simulink model "scc_ut"  (Simulink 8.1)
settings: Solver=FixedStepDiscrete  StartTime=0.0  StopTime=10  FixedStep=5E-3  RelTol=1e-3
PostLoadFcn:
  | , if any(exist('dsrtsu_mdlpostloadfcn', 'file') == [2, 3, 6]), try dsrtsu_mdlpostloadfcn('Execute', bdroot); catch fprintf('Error in PostLoadFcn (dsrtsu_mdlpostloadfcn) for model "%s":\n %s\n', bdroot, lasterr); end, end,
libraries: siltestlib x20, scc x1
settings Model: DSRTSU_INTERNAL_RTI_VER=450  DSRTSU_INTERNAL_RTI_TYPE=rti1401  RTICANMMDATA=struct('GeneralSetupData',struct('modelroot','D:\ELN150201_TAIWAN\trunk\AdasDragon\software\sw_development\arch\app\acc','generalsettings',struct('filesettings',struct('destfolder',struct('Name','RTICANMM_FILES','Check',1),'buildfolder',struct('Name','.','Check',1),'AbsDestfolder',struct('Name','D:\ELN150201_TAIWAN\trunk\AdasDragon\software\sw_development\arch\app\acc\RTICANMM_FILES'),'AbsBuildfolder',struct('Name','D:\ELN150201_TAIWAN\trunk\AdasDragon\software\sw_development\arch\app\acc'))),'options',struct('addpaths',1,'rmpaths',1,'addtrcexclusion',logical(1),'cannavigator',struct('checkmonitoring',0),'show_usrtrc',0,'use_usrtrc',0),'advanced',struct('options',[1 1 1 1 1 1 1 1 1 1 1 1 1 1 1 1 1 1 1 1 1 1 1 1 1 1 1 1 1 1 1 1 1 1 1 1 1 1 1 1 1 1 1 1 1 1 1 1 1 1 1 1 1 1 1 1 1 1 1 1 1 1 1 1 1 1 1 1 1 1 1 1 1 1 1 1 1 1 1 1 1 1 1 1 1 1 1 1 1 1 1 1 1 1 1 1 1 1 1 1]),'MPSetup',{{}},'modelname','scc_ut','block','scc_ut'))  DSRTSU_INTERNAL_RTIFPGA=40  Creator=AT015411  LastModifiedBy=AT015555  BufferReuse=off
settings DataIOCC: SignalLoggingSaveFormat=Dataset
settings OptimizationCC: BlockReduction=off  OptimizeBlockIOStorage=off  BufferReuse=off  ExpressionFolding=off  ExpressionDepthLimit=128  LocalBlockOutputs=off
settings DebuggingCC: FcnCallInpInsideContextMsg=EnableAllAsError
settings HardwareCC: ProdIntDivRoundTo=Zero  ProdEndianess=BigEndian  ProdHWDeviceType=Generic->Custom  TargetIntDivRoundTo=Zero  TargetEndianess=BigEndian  TargetHWDeviceType=Generic->Custom
settings RTWCC: SystemTargetFile=rti1005.tlc  MakeCommand=make_rti  TemplateMakefile=rti1005.tmf  Description=dSPACE DS1005 Hardware Platform  ProcessScript=rti1005_make_rtw_hook
settings STFCustomTargetCC: CodeReplacementLibrary=ANSI_C  ParMdlRefBuildCompliant=on  GeneratePreprocessorConditionals=Disable all  MatFileLogging=on  SystemTargetFile=rti1005.tlc
settings GRTTargetCC: CompOptLevelCompliant=off  ConcurrentExecutionCompliant=off  ExtModeMexFile=noextcomm
settings CustomProperty: DataType=RTWOptions_EnumType_C__Program Files (x86)_dSPACE RCPHIL 2014-B_MATLAB_RTI_RTI1401_TLC_rti1005_1InitialSimState  Value=RUN
settings EnumStrPairs: String=RUN

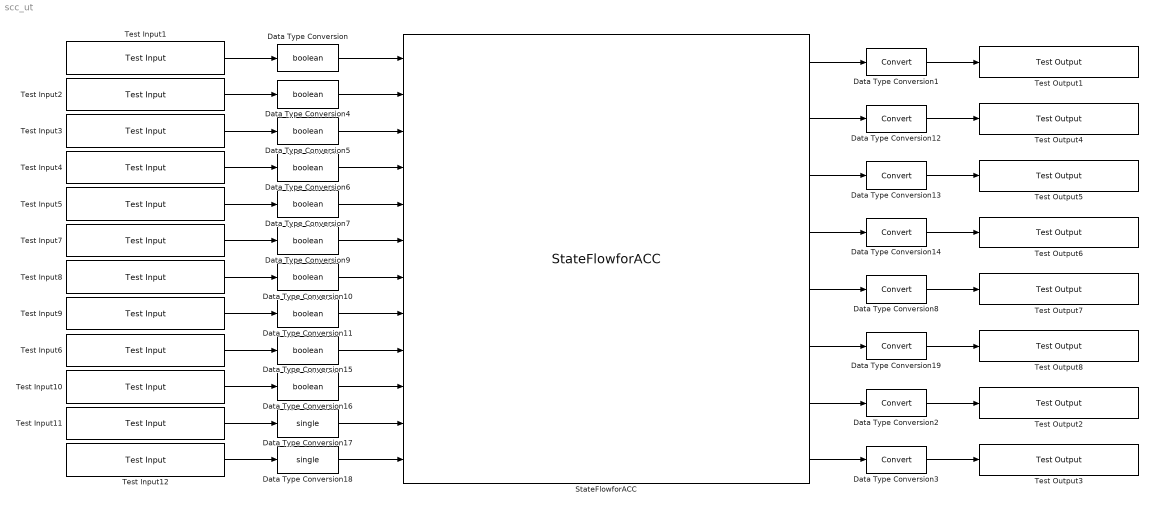
== system scc_ut ==
  Data Type Conversion{,4..7,9..11,15..16} (10 alike) : DataTypeConversion  OutDataTypeStr=boolean
  Data Type Conversion{1..3,8,12..14,19} (8 alike) : DataTypeConversion
  Data Type Conversion17 : DataTypeConversion  OutDataTypeStr=single
  Data Type Conversion18 : DataTypeConversion  OutDataTypeStr=single
  StateFlowforACC : scc/StateFlowforACC
  Test Input1 : siltestlib/Test Input  varname=VIFO_ACCTurnOnReq_flg  sampletime=0.005
  Test Input10 : siltestlib/Test Input  varname=VACC_ACCHoldReqDisablePrev_flg  sampletime=0.005
  Test Input11 : siltestlib/Test Input  varname=VIFO_ACCVehClearance_m  sampletime=0.005
  Test Input12 : siltestlib/Test Input  varname=KACC_DefStandstillClearance_m  sampletime=0.005
  Test Input2 : siltestlib/Test Input  varname=VIFO_ACCTurnOffReq_flg  sampletime=0.005
  Test Input3 : siltestlib/Test Input  varname=VJUD_ACCEnableReq_flg  sampletime=0.005
  Test Input4 : siltestlib/Test Input  varname=VJUD_ACCActiveReq_flg  sampletime=0.005
  Test Input5 : siltestlib/Test Input  varname=VJUD_ACCDeactivationReq_flg  sampletime=0.005
  Test Input6 : siltestlib/Test Input  varname=VACC_ACCHoldReqEnablePrev_flg  sampletime=0.005
  Test Input7 : siltestlib/Test Input  varname=VJUD_ACCStandstillReq_flg  sampletime=0.005
  Test Input8 : siltestlib/Test Input  varname=VJUD_ACCRefollowReq_flg  sampletime=0.005
  Test Input9 : siltestlib/Test Input  varname=VJUD_ACCOverrideReq_flg  sampletime=0.005
  Test Output1 : siltestlib/Test Output  varname=VACC_ACCStateHMI_enum  sampletime=-1
  Test Output2 : siltestlib/Test Output  varname=VACC_ACCActing_flg  sampletime=-1
  Test Output3 : siltestlib/Test Output  varname=VACC_ACCOverride_flg  sampletime=-1
  Test Output4 : siltestlib/Test Output  varname=VACC_ACCSystemState_enum  sampletime=-1
  Test Output5 : siltestlib/Test Output  varname=VACC_ACCTqReqAppl_flg  sampletime=-1
  Test Output6 : siltestlib/Test Output  varname=VACC_ACCDecelReqAppl_flg  sampletime=-1
  Test Output7 : siltestlib/Test Output  varname=VACC_ACCHoldReq_flg  sampletime=-1
  Test Output8 : siltestlib/Test Output  varname=VACC_StandstillClearance_m  sampletime=-1
  wires:
  Data Type Conversion1/1 -> Test Output1/1
  Test Input1/1 -> Data Type Conversion/1
  StateFlowforACC/1 -> Data Type Conversion1/1
  Data Type Conversion2/1 -> Test Output2/1
  Data Type Conversion3/1 -> Test Output3/1
  Test Input2/1 -> Data Type Conversion4/1
  Test Input3/1 -> Data Type Conversion5/1
  Test Input4/1 -> Data Type Conversion6/1
  Test Input5/1 -> Data Type Conversion7/1
  Test Input7/1 -> Data Type Conversion9/1
  Test Input8/1 -> Data Type Conversion10/1
  Test Input9/1 -> Data Type Conversion11/1
  Data Type Conversion7/1 -> StateFlowforACC/5
  Data Type Conversion6/1 -> StateFlowforACC/4
  Data Type Conversion5/1 -> StateFlowforACC/3
  Data Type Conversion4/1 -> StateFlowforACC/2
  Data Type Conversion/1 -> StateFlowforACC/1
  Data Type Conversion12/1 -> Test Output4/1
  Data Type Conversion13/1 -> Test Output5/1
  Data Type Conversion14/1 -> Test Output6/1
  StateFlowforACC/2 -> Data Type Conversion12/1
  StateFlowforACC/3 -> Data Type Conversion13/1
  StateFlowforACC/4 -> Data Type Conversion14/1
  Data Type Conversion9/1 -> StateFlowforACC/6
  Data Type Conversion10/1 -> StateFlowforACC/7
  Data Type Conversion11/1 -> StateFlowforACC/8
  Data Type Conversion8/1 -> Test Output7/1
  StateFlowforACC/5 -> Data Type Conversion8/1
  Test Input6/1 -> Data Type Conversion15/1
  Test Input10/1 -> Data Type Conversion16/1
  Data Type Conversion15/1 -> StateFlowforACC/9
  Data Type Conversion16/1 -> StateFlowforACC/10
  Test Input11/1 -> Data Type Conversion17/1
  Test Input12/1 -> Data Type Conversion18/1
  Data Type Conversion17/1 -> StateFlowforACC/11
  Data Type Conversion18/1 -> StateFlowforACC/12
  Data Type Conversion19/1 -> Test Output8/1
  StateFlowforACC/6 -> Data Type Conversion19/1
  StateFlowforACC/7 -> Data Type Conversion2/1
  StateFlowforACC/8 -> Data Type Conversion3/1
